simulink model "TangapCumdongluc_2023b"  (R2023b)
settings: Solver=FixedStepAuto  StartTime=0  StopTime=43.98  FixedStep=0.00025  RelTol=1e-3  AbsTol=1e-3  EnableMultiTasking=on
undefined symbols (not defined in the file): h, km, Lm, m, rad, Rm, s
libraries: aerolibconvert2 x2, SignalEditorBlockLib x1
settings Model: Creator=Admin  LastModifiedBy=Legion
settings SolverCC: AutoScaleAbsTol=off  AlgebraicLoopSolver=TrustRegion  MaxZcPerStep=1
settings DataIOCC: LimitDataPoints=on  MaxDataPoints=10000
settings OptimizationCC: ReuseModelBlockBuffer=off  LifeSpan=inf
settings DebuggingCC: UnconnectedInputMsg=warning  UnconnectedOutputMsg=warning  UnconnectedLineMsg=warning  AllowSymbolicDim=off  SubsystemReferenceDiagnosticForUnitTest=warning  SFUnexpectedBacktrackingDiag=warning  SFNoUnconditionalDefaultTransitionDiag=warning  SFExecutionAtInitializationDiag=none  ArithmeticOperatorsInVariantConditions=warning
settings ModelReferenceCC: EnableRefExpFcnMdlSchedulingChecks=on
settings SFSimCC: SimUseLocalCustomCode=off  CustomCodeUndefinedFunction=UseInterfaceOnly
settings RTWCC: RTWUseLocalCustomCode=off  DLArmComputeVersion=19.05
settings CodeAppCC: StateflowObjectComments=on
settings GRTTargetCC: TargetLangStandard=C89/C90 (ANSI)
settings ConfigComp: CovMetricSettings=dw  CovSaveCumulativeToWorkspaceVar=on  CovSaveSingleToWorkspaceVar=on  CovExternalEMLEnable=off  CovSFcnEnable=off
settings SimscapeCC: SimscapeLogType=all  SimscapeLogSimulationStatistics=on  SimscapeLogDataHistory=10000

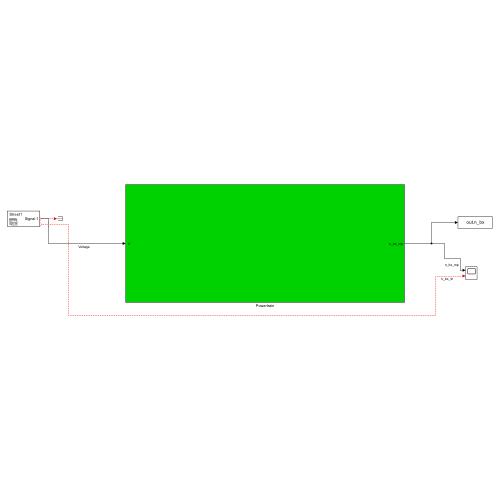
[thumbnail: Simulink's stored preview of the top-level diagram]
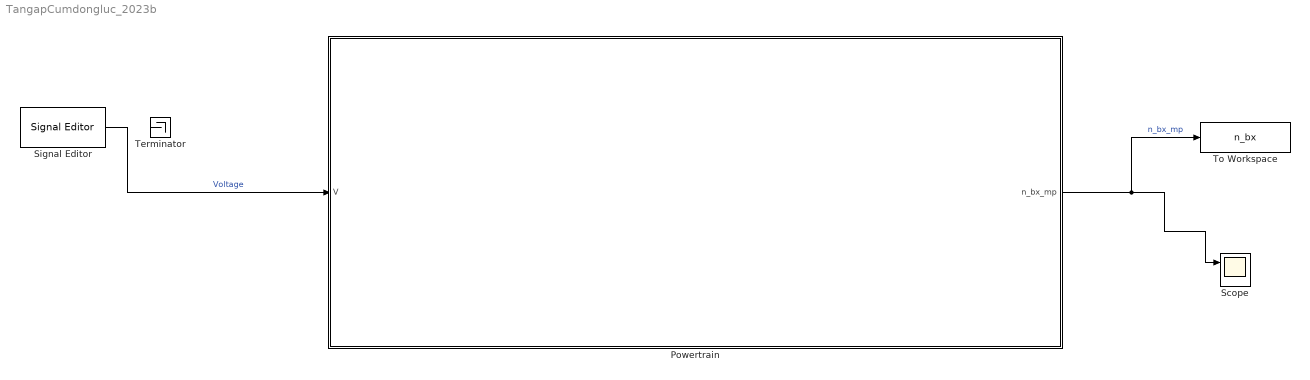
== system TangapCumdongluc_2023b ==
  Powertrain : Subsystem
  Scope : Scope  NumInputPorts=2
  Signal Editor : SignalEditorBlockLib/Signal Editor  FileName=DataTangapcumdongluc.mat  ActiveScenario=Sheet1  ActiveSignal=Voltage  IsBus=off  OutputBusObjectStr=Bus: BusObject  SampleTime=0  ZeroCross=off  OutputAfterFinalValue=Setting to zero  Unit=inherit  PreserveSignalName=on  ApplySigPropsToAllScenarios=on  ApplySigPropsToAllSignals=off
  Terminator : Terminator
  To Workspace : ToWorkspace  VariableName=n_bx  SaveFormat=Timeseries  SampleTime=-1
  wires:
  Signal Editor/1 -> Powertrain/1(" V")  "Voltage"
  Powertrain/1(n_bx_mp) -> To Workspace/1, Scope/1  "n_bx_mp"
  ? -> Scope/2  "n_bx_tn"
  ? -> Terminator/1

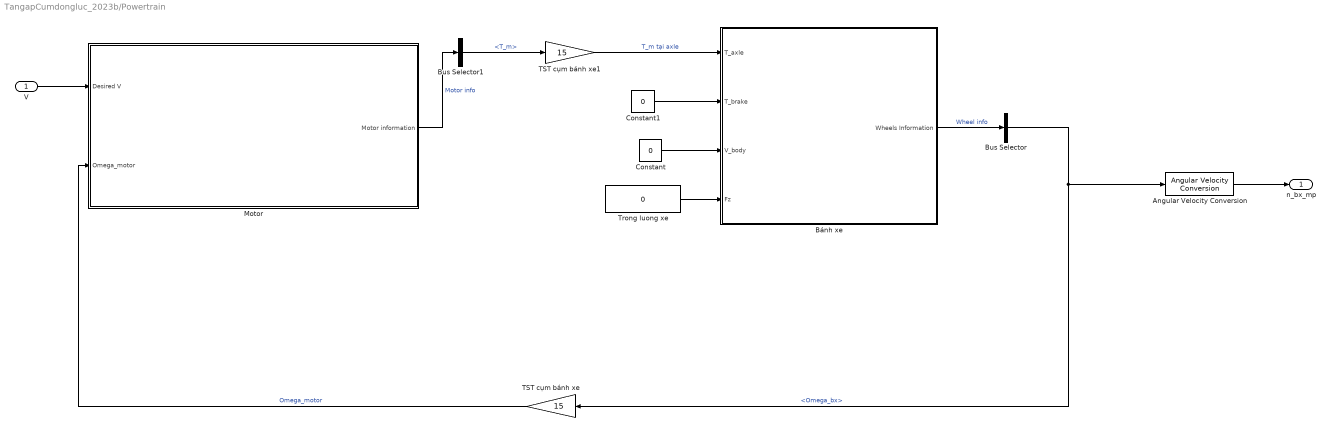
== system TangapCumdongluc_2023b/Powertrain ==
  " V" : Inport
  Angular Velocity Conversion : aerolibconvert2/Angular Velocity Conversion  IU=rad/s  OU=rpm
  Bus Selector : BusSelector  OutputSignals=Omega_bx
  Bus Selector1 : BusSelector  OutputSignals=T_m
  Bánh xe : Subsystem
  Constant : Constant  Value=0
  Constant1 : Constant  Value=0
  Motor : Subsystem
  TST cụm bánh xe : Gain  Gain=15
  TST cụm bánh xe1 : Gain  Gain=15
  Trong luong xe : Constant  Value=0
  n_bx_mp : Outport
  wires:
  Bánh xe/1(Wheels Information) -> Bus Selector/1  "Wheel info"
  " V"/1 -> Motor/1(" Desired V")
  Bus Selector1/1 -> TST cụm bánh xe1/1  "<T_m>"
  TST cụm bánh xe1/1 -> Bánh xe/1(T_axle)  "T_m tại axle"
  TST cụm bánh xe/1 -> Motor/2(Omega_motor)  "Omega_motor"
  Trong luong xe/1 -> Bánh xe/4(Fz)
  Constant1/1 -> Bánh xe/2(T_brake)
  Bus Selector/1 -> Angular Velocity Conversion/1, TST cụm bánh xe/1  "<Omega_bx>"
  Motor/1(Motor information) -> Bus Selector1/1  "Motor info"
  Angular Velocity Conversion/1 -> n_bx_mp/1
  Constant/1 -> Bánh xe/3(V_body)

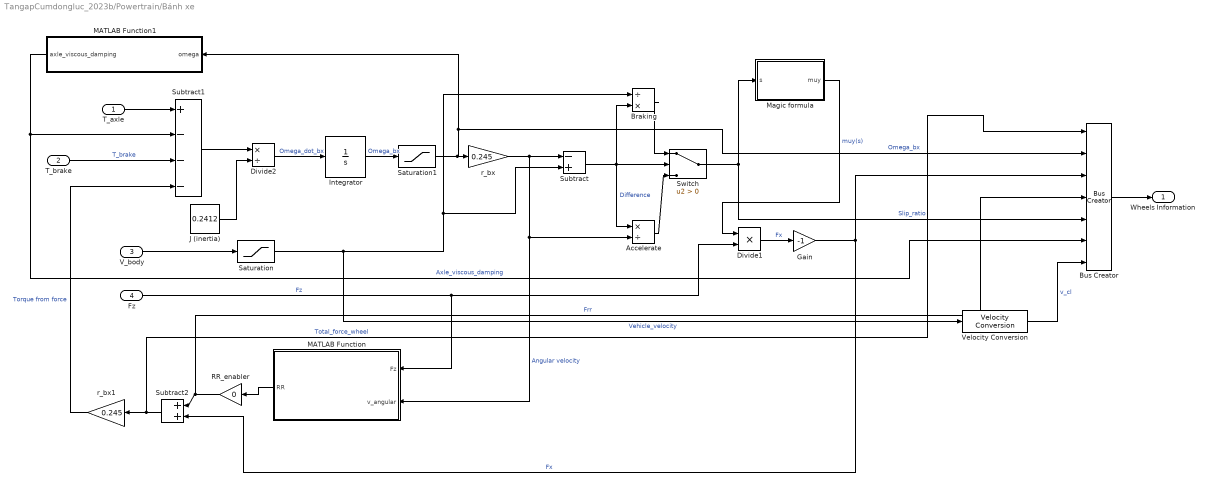
== system TangapCumdongluc_2023b/Powertrain/Bánh xe ==
  T_axle : Inport
  T_brake : Inport  Port=2
  V_body : Inport  Port=3
  Fz : Inport  Port=4
  Accelerate : Product  Inputs=*/
  Braking : Product  Inputs=/*
  Bus Creator : BusCreator  Inputs=7
  Divide1 : Product  Inputs=**
  Divide2 : Product  Inputs=*/
  Gain : Gain  Gain=-1
  Integrator : Integrator  LimitOutput=on  LowerSaturationLimit=0
  J (inertia) : Constant  Value=0.2412
  MATLAB Function : MATLAB Function  TreatAsAtomicUnit=on
  MATLAB Function1 : MATLAB Function  TreatAsAtomicUnit=on
  Magic formula : MATLAB Function  TreatAsAtomicUnit=on
  RR_enabler : Gain  Gain=0
  Saturation : Saturate  UpperLimit=inf  LowerLimit=0.00000000000000001
  Saturation1 : Saturate  UpperLimit=inf  LowerLimit=0.00000000000000001  ZeroCross=off
  Subtract : Sum  Inputs=-+
  Subtract1 : Sum  Inputs=+---
  Subtract2 : Sum
  Switch : Switch  Criteria=u2 > Threshold  SaturateOnIntegerOverflow=off  InputSameDT=off
  Velocity Conversion : aerolibconvert2/Velocity Conversion  IU=m/s  OU=km/h
  r_bx : Gain  Gain=0.245
  r_bx1 : Gain  Gain=0.245
  Wheels Information : Outport
  wires:
  Fz/1 -> Divide1/2, MATLAB Function/1(Fz)  "Fz"
  Subtract/1 -> Switch/2, Accelerate/1, Braking/2  "Difference"
  Saturation/1 -> Velocity Conversion/1, Braking/1, Subtract/2  "Vehicle_velocity"
  T_axle/1 -> Subtract1/1
  T_brake/1 -> Subtract1/3  "T_brake"
  Magic formula/1(muy) -> Divide1/1  "muy(s)"
  Accelerate/1 -> Switch/3
  Braking/1 -> Switch/1
  Switch/1 -> Bus Creator/5, Magic formula/1(s)  "Slip_ratio"
  Subtract1/1 -> Divide2/1
  J (inertia)/1 -> Divide2/2
  Divide2/1 -> Integrator/1  "Omega_dot_bx"
  Divide1/1 -> Gain/1  "Fx"
  Gain/1 -> Bus Creator/3, Subtract2/2  "Fx"
  V_body/1 -> Saturation/1
  r_bx/1 -> Subtract/1, Accelerate/2, MATLAB Function/2(v_angular)  "Angular velocity"
  RR_enabler/1 -> Bus Creator/4, Subtract2/1  "Frr"
  MATLAB Function/1(RR) -> RR_enabler/1
  Subtract2/1 -> Bus Creator/1, r_bx1/1  "Total_force_wheel"
  r_bx1/1 -> Subtract1/4  "Torque from force"
  Saturation1/1 -> Bus Creator/2, MATLAB Function1/1(omega), r_bx/1  "Omega_bx"
  MATLAB Function1/1(axle_viscous_damping) -> Subtract1/2, Bus Creator/6  "Axle_viscous_damping"
  Integrator/1 -> Saturation1/1  "Omega_bx"
  Bus Creator/1 -> Wheels Information/1
  Velocity Conversion/1 -> Bus Creator/7  "v_cl"

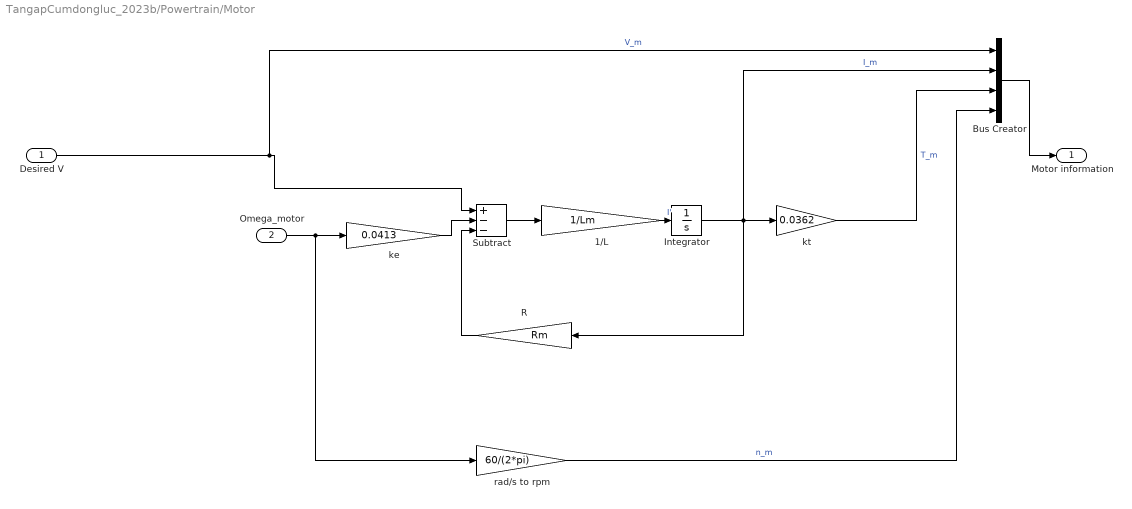
== system TangapCumdongluc_2023b/Powertrain/Motor ==
  " Desired V" : Inport
  Omega_motor : Inport  Port=2
  1/L : Gain  Gain=1/Lm
  Bus Creator : BusCreator  Inputs=4
  Integrator : Integrator
  R : Gain  Gain=Rm
  Subtract : Sum  Inputs=+--
  ke : Gain  Gain=0.0413
  kt : Gain  Gain=0.0362
  rad/s to rpm : Gain  Gain=60/(2*pi)
  Motor information : Outport
  wires:
  Omega_motor/1 -> rad/s to rpm/1, ke/1
  R/1 -> Subtract/3
  ke/1 -> Subtract/2
  Subtract/1 -> 1/L/1
  1/L/1 -> Integrator/1  "I'"
  Integrator/1 -> Bus Creator/2, R/1, kt/1  "I_m"
  Bus Creator/1 -> Motor information/1
  " Desired V"/1 -> Subtract/1, Bus Creator/1  "V_m"
  kt/1 -> Bus Creator/3  "T_m"
  rad/s to rpm/1 -> Bus Creator/4  "n_m"

== matlab function TangapCumdongluc_2023b/Powertrain/Bánh xe/Magic formula ==
  data: s input; muy output
function muy = magicformula(s)
% Khai báo hằng số mặt đường
B = 10;
C = 1.65;
D = 1;
E = 0.01;
% Magic formula
muy = D * sin(C * atan(B * s - E * (B * s - atan(B * s))));

== matlab function TangapCumdongluc_2023b/Powertrain/Bánh xe/MATLAB Function1 ==
  data: omega input; axle_viscous_damping output
function axle_viscous_damping = fcn(omega)
    axle_viscous_damping=0.0362*(0.2657*(omega)+6.7129)*15;

== matlab function TangapCumdongluc_2023b/Powertrain/Bánh xe/MATLAB Function ==
  data: Fz input; RR output; v_angular input
function RR = rolling_resistance_function(Fz,v_angular)

RR = (0.015+7*10^(-6)*v_angular^2)*Fz;
